simulink model "Vehicle"  (R2013a)
settings: Solver=ode45  StartTime=0.0  StopTime=10.0  RelTol=1e-3
settings Model: Creator=Nathan  LastModifiedBy=Nathan
settings SolverCC: ZeroCrossControl=DisableAll
settings OptimizationCC: InlineParams=on

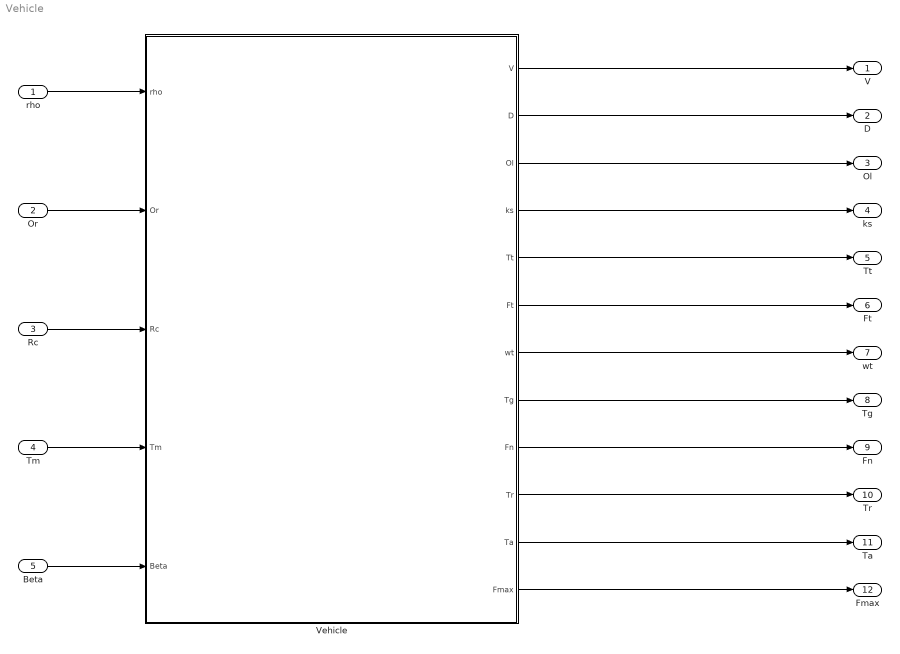
== system Vehicle ==
  rho : Inport
  Or : Inport  Port=2
  Rc : Inport  Port=3
  Tm : Inport  Port=4
  Beta : Inport  Port=5
  Vehicle : Subsystem
  V : Outport
  D : Outport  Port=2
  Ol : Outport  Port=3
  ks : Outport  Port=4
  Tt : Outport  Port=5
  Ft : Outport  Port=6
  wt : Outport  Port=7
  Tg : Outport  Port=8
  Fn : Outport  Port=9
  Tr : Outport  Port=10
  Ta : Outport  Port=11
  Fmax : Outport  Port=12
  wires:
  Vehicle/1(V) -> V/1
  Vehicle/2(D) -> D/1
  Vehicle/3(Ol) -> Ol/1
  Vehicle/4(ks) -> ks/1
  Vehicle/5(Tt) -> Tt/1
  Vehicle/6(Ft) -> Ft/1
  Vehicle/7(wt) -> wt/1
  Vehicle/8(Tg) -> Tg/1
  Vehicle/9(Fn) -> Fn/1
  Vehicle/10(Tr) -> Tr/1
  Vehicle/11(Ta) -> Ta/1
  Vehicle/12("Fmax ") -> Fmax/1
  rho/1 -> Vehicle/1(rho)
  Or/1 -> Vehicle/2(Or)
  Rc/1 -> Vehicle/3(Rc)
  Tm/1 -> Vehicle/4(Tm)
  Beta/1 -> Vehicle/5(Beta)

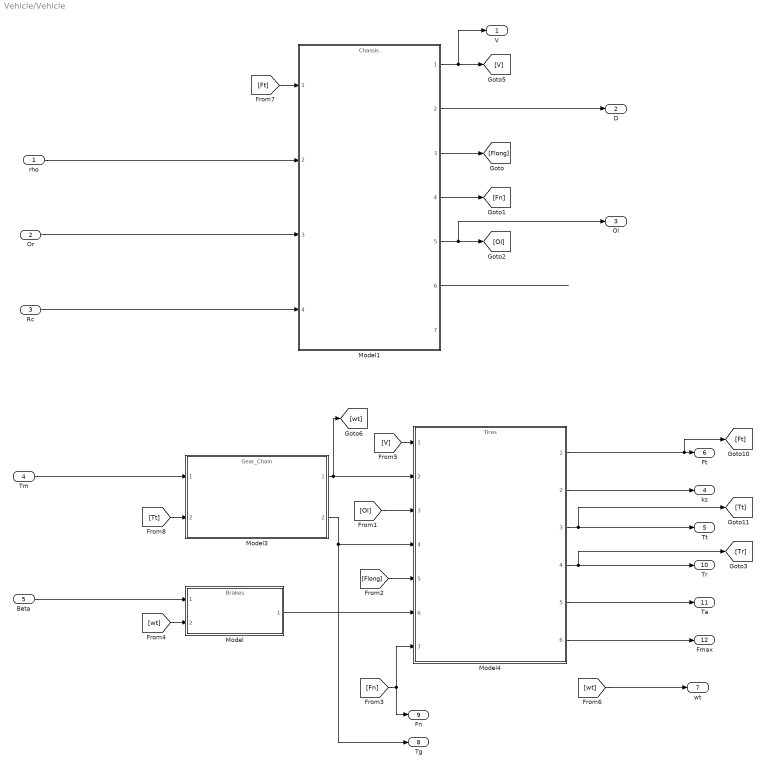
== system Vehicle/Vehicle ==
  rho : Inport
  Or : Inport  Port=2
  Rc : Inport  Port=3
  Tm : Inport  Port=4
  Beta : Inport  Port=5
  Model : ModelReference  ModelNameDialog=Brakes.slx  SimulationMode=Normal  ModelReferenceVersion=1.5  CopyOfModelName=Brakes.slx  DefaultDataLogging=on
  Model1 : ModelReference  ModelNameDialog=Chassis.slx  SimulationMode=Normal  ModelReferenceVersion=1.16  CopyOfModelName=Chassis.slx  DefaultDataLogging=on
  Model3 : ModelReference  ModelNameDialog=Gear_Chain.slx  SimulationMode=Normal  ModelReferenceVersion=1.15  CopyOfModelName=Gear_Chain.slx  DefaultDataLogging=on
  Model4 : ModelReference  ModelNameDialog=Tires.slx  SimulationMode=Normal  ModelReferenceVersion=1.77  CopyOfModelName=Tires.slx  DefaultDataLogging=on
  V : Outport
  D : Outport  Port=2
  Ol : Outport  Port=3
  ks : Outport  Port=4
  Tt : Outport  Port=5
  Ft : Outport  Port=6
  wt : Outport  Port=7
  Tg : Outport  Port=8
  Fn : Outport  Port=9
  Tr : Outport  Port=10
  Ta : Outport  Port=11
  "Fmax " : Outport  Port=12
  wires:
  Model1/3 -> [Flong]
  [Ol] -> Model4/3
  Model1/4 -> [Fn]
  Model1/5 -> Ol/1, [Ol]
  Model3/1 -> Model4/2, [wt]
  [Tt] -> Model3/2
  [Ft] -> Model1/1
  Model3/2 -> Tg/1, Model4/4
  [wt] -> Model/2
  [V] -> Model4/1
  [Fn] -> Model4/7, Fn/1
  Model1/1 -> V/1, [V]
  [Flong] -> Model4/5
  Model1/6 -> ?
  Or/1 -> Model1/3
  Beta/1 -> Model/1
  Tm/1 -> Model3/1
  Rc/1 -> Model1/4
  rho/1 -> Model1/2
  Model4/1 -> Ft/1, [Ft]
  [wt] -> wt/1
  Model/1 -> Model4/6
  Model1/2 -> D/1
  Model4/2 -> ks/1
  Model4/3 -> [Tt], Tt/1
  Model4/4 -> [Tr], Tr/1
  Model4/5 -> Ta/1
  Model4/6 -> "Fmax "/1
